simulink model "sl_MCD_sincrono"  (R2016b)
settings: Solver=VariableStepAuto  StartTime=0.0  StopTime=t_sim  RelTol=1e-3
values from neighbouring files (symbols this model uses):
  ampl_sin = input(selection)    [pruebas_MCD.m]
  freq = input(selection)    [pruebas_MCD.m]
  omega = 0    [pruebas_MCD.m]
  omega_sat = [-0.2618 0.2618]    [pruebas_MCD.m]    (also in pruebas_MCI.m = [-0.2618/10 0.2618/10])
  pos_init = [0;0;0]    [pruebas_MCD.m]    (also in pruebas_MCI.m = [0;0;0.2915])
  sel = input(selection)    [pruebas_MCD.m]
  tetha_d = tetha_d_sat(1)    [pruebas_MCD.m]
  tetha_d_sat = [-0.75 0.75]    [pruebas_MCD.m]    (also in pruebas_MCI.m = [-0.75/2 0.75/2])
settings Model: Creator=marrcogrova  LastModifiedBy=Javi Owo

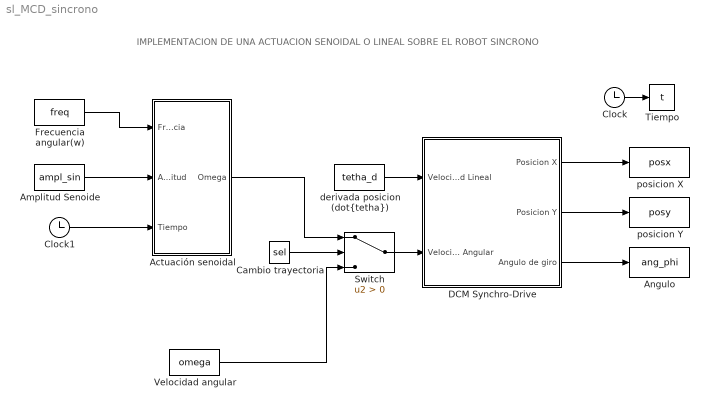
== system sl_MCD_sincrono ==
  note: IMPLEMENTACION DE UNA ACTUACION SENOIDAL
      | O LINEAL SOBRE EL ROBOT SINCRONO
  Actuación senoidal : Subsystem
  "Amplitud Senoide " : Constant  Value=ampl_sin
  Angulo : ToWorkspace  VariableName=ang_phi  SampleTime=-1
  Cambio trayectoria : Constant  Value=sel
  Clock : Clock
  Clock1 : Clock
  DCM Synchro-Drive : Subsystem
  Frecuencia angular(w) : Constant  Value=freq
  Switch : Switch  Criteria=u2 > Threshold
  Tiempo : ToWorkspace  VariableName=t  SampleTime=-1
  Velocidad angular : Constant  Value=omega
  "derivada posicion (dot{tetha})" : Constant  Value=tetha_d
  posicion X : ToWorkspace  VariableName=posx  SampleTime=-1
  posicion Y : ToWorkspace  VariableName=posy  SampleTime=-1
  wires:
  DCM Synchro-Drive/3(Angulo de giro) -> Angulo/1
  Clock/1 -> Tiempo/1
  "derivada posicion (dot{tetha})"/1 -> DCM Synchro-Drive/1(Velocidad Lineal)
  Clock1/1 -> Actuación senoidal/3(Tiempo)
  Frecuencia angular(w)/1 -> Actuación senoidal/1("Frecuencia ")
  "Amplitud Senoide "/1 -> Actuación senoidal/2("Amplitud ")
  DCM Synchro-Drive/1(Posicion X) -> posicion X/1
  DCM Synchro-Drive/2(Posicion Y) -> posicion Y/1
  Switch/1 -> DCM Synchro-Drive/2(Velocidad Angular)
  Actuación senoidal/1(Omega) -> Switch/1
  Velocidad angular/1 -> Switch/3
  Cambio trayectoria/1 -> Switch/2

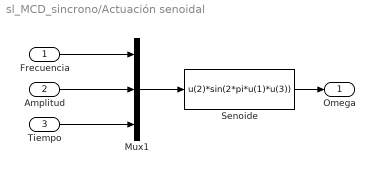
== system sl_MCD_sincrono/Actuación senoidal ==
  "Frecuencia " : Inport
  "Amplitud " : Inport  Port=2
  Tiempo : Inport  Port=3
  Mux1 : Mux  Inputs=3
  Senoide : Fcn  Expr=u(2)*sin(2*pi*u(1)*u(3))
  Omega : Outport
  wires:
  Senoide/1 -> Omega/1
  "Frecuencia "/1 -> Mux1/1
  Mux1/1 -> Senoide/1
  "Amplitud "/1 -> Mux1/2
  Tiempo/1 -> Mux1/3

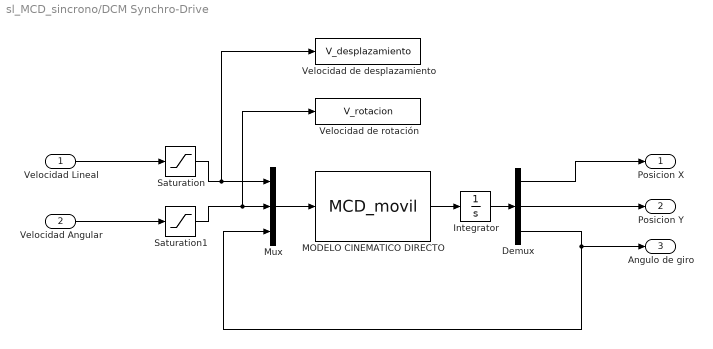
== system sl_MCD_sincrono/DCM Synchro-Drive ==
  Velocidad Lineal : Inport
  Velocidad Angular : Inport  Port=2
  Demux : Demux  Outputs=3
  Integrator : Integrator  InitialCondition=pos_init
  MODELO CINEMATICO DIRECTO : MATLABFcn  MATLABFcn=MCD_movil  OutputDimensions=3
  Mux : Mux  Inputs=3
  Saturation : Saturate  UpperLimit=tetha_d_sat(2)  LowerLimit=tetha_d_sat(1)
  Saturation1 : Saturate  UpperLimit=omega_sat(2)  LowerLimit=omega_sat(1)
  Velocidad de desplazamiento : ToWorkspace  VariableName=V_desplazamiento  SaveFormat=Timeseries  SampleTime=-1
  Velocidad de rotación : ToWorkspace  VariableName=V_rotacion  SaveFormat=Timeseries  SampleTime=-1
  Posicion X : Outport
  Posicion Y : Outport  Port=2
  Angulo de giro : Outport  Port=3
  wires:
  Integrator/1 -> Demux/1
  Demux/3 -> Angulo de giro/1, Mux/3
  Demux/1 -> Posicion X/1
  Demux/2 -> Posicion Y/1
  Mux/1 -> MODELO CINEMATICO DIRECTO/1
  MODELO CINEMATICO DIRECTO/1 -> Integrator/1
  Velocidad Lineal/1 -> Saturation/1
  Saturation/1 -> Velocidad de desplazamiento/1, Mux/1
  Saturation1/1 -> Velocidad de rotación/1, Mux/2
  Velocidad Angular/1 -> Saturation1/1
